simulink model "Complementary_Filter"  (R2025a)
settings: Solver=VariableStepAuto  StartTime=0.0  StopTime=10.0  RelTol=1e-3
settings Model: Creator=xing2  LastModifiedBy=xing2

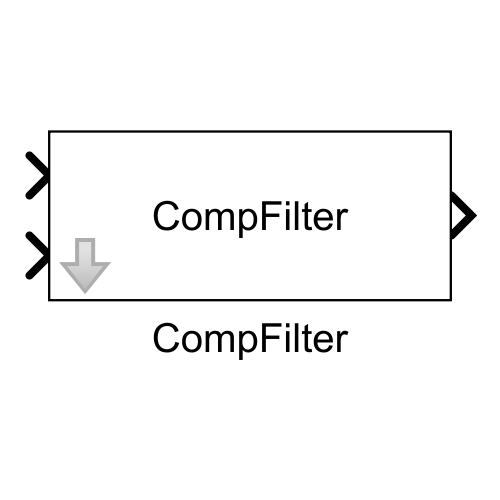
[thumbnail: Simulink's stored preview of the top-level diagram]
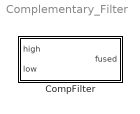
== system Complementary_Filter ==
  CompFilter : Subsystem  mask{alpha=0.98}
      mask prompts: alpha "alpha (0~1)"
      mask help: Complementary Filter: alpha*high + (1-alpha)*low
      mask Display: disp('CompFilter');

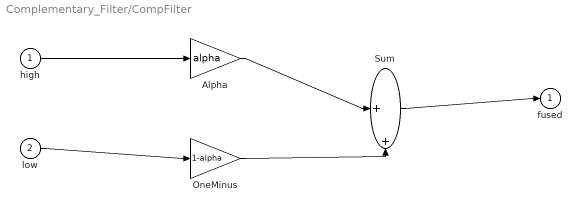
== system Complementary_Filter/CompFilter ==
  high : Inport
  low : Inport  Port=2
  Alpha : Gain  Gain=alpha
  OneMinus : Gain  Gain=1-alpha
  Sum : Sum  Inputs=|++
  fused : Outport
  wires:
  high/1 -> Alpha/1
  low/1 -> OneMinus/1
  Alpha/1 -> Sum/1
  OneMinus/1 -> Sum/2
  Sum/1 -> fused/1
